simulink library "Test_lib"  (R2023b)
settings: Solver=VariableStepAuto  StartTime=0.0  StopTime=10.0  RelTol=1e-3
settings Model: Creator=FIRSTMentor  LastModifiedBy=hilat

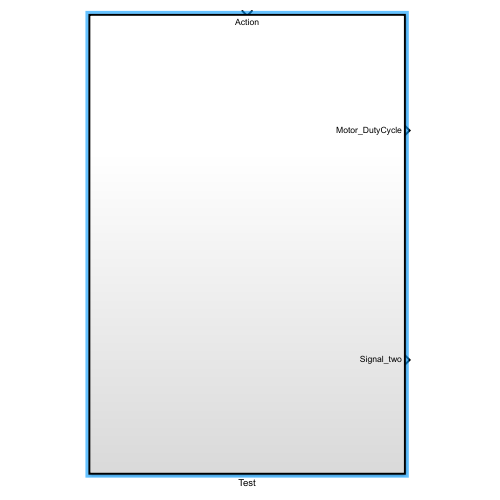
[thumbnail: Simulink's stored preview of the top-level diagram]
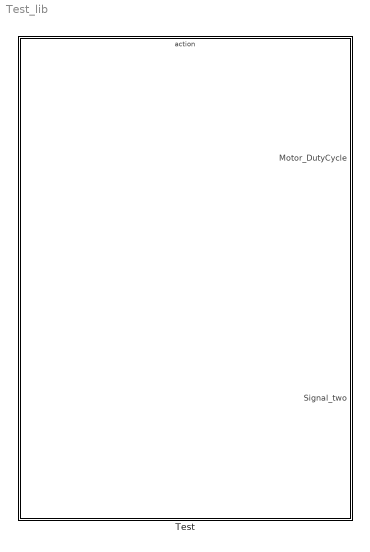
== system Test_lib ==
  Test : Subsystem  TreatAsAtomicUnit=on

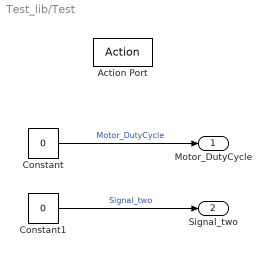
== system Test_lib/Test ==
  Action Port : ActionPort  InitializeStates=reset
  Constant : Constant  Value=0
  Constant1 : Constant  Value=0
  Motor_DutyCycle : Outport
  Signal_two : Outport  Port=2
  wires:
  Constant1/1 -> Signal_two/1  "Signal_two"
  Constant/1 -> Motor_DutyCycle/1  "Motor_DutyCycle"
